simulink model "quadrotor_modules"  (R2020b)
settings: Solver=VariableStepAuto  StartTime=0.0  StopTime=10.0  RelTol=1e-3
values from neighbouring files (symbols this model uses):
  b = 1    [quadrotor_parameters.m]
  d = 1    [quadrotor_parameters.m]
  g = 9.81    [quadrotor_parameters.m]
  Ix = 1    [quadrotor_parameters.m]
  Iy = 1    [quadrotor_parameters.m]
  Iz = 1.5    [quadrotor_parameters.m]
  l = 1    [quadrotor_parameters.m]
  m = 1    [quadrotor_parameters.m]
settings Model: Creator=Алексей  LastModifiedBy=Алексей

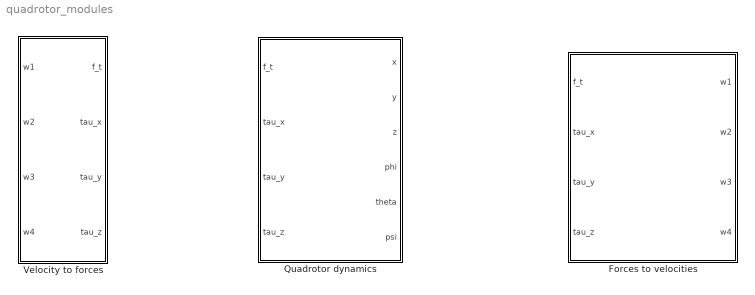
== system quadrotor_modules ==
  Forces to velocities : Subsystem
  Quadrotor dynamics : Subsystem
  Velocity to forces : Subsystem

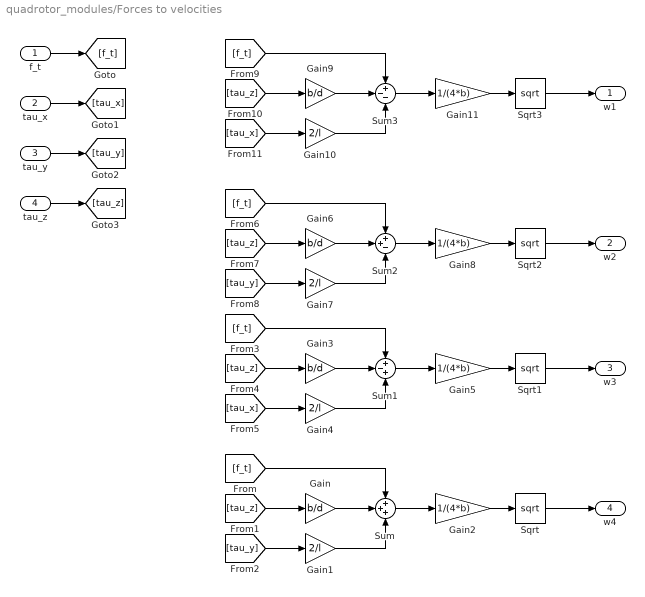
== system quadrotor_modules/Forces to velocities ==
  f_t : Inport
  tau_x : Inport  Port=2
  tau_y : Inport  Port=3
  tau_z : Inport  Port=4
  Gain{,3,6,9} (4 alike) : Gain  Gain=b/d
  Gain{1,4,7,10} (4 alike) : Gain  Gain=2/l
  Gain{2,5,8,11} (4 alike) : Gain  Gain=1/(4*b)
  Sqrt{,1..3} (4 alike) : Sqrt  SaturateOnIntegerOverflow=on
  Sum : Sum  Inputs=+++
  Sum1 : Sum  Inputs=+-+
  Sum2 : Sum  Inputs=++-
  Sum3 : Sum  Inputs=+--
  w1 : Outport
  w2 : Outport  Port=2
  w3 : Outport  Port=3
  w4 : Outport  Port=4
  wires:
  f_t/1 -> [f_t]
  [tau_y] -> Gain1/1
  [f_t] -> Sum/1
  Gain2/1 -> Sqrt/1
  Sqrt/1 -> w4/1
  Sum/1 -> Gain2/1
  tau_x/1 -> [tau_x]
  Gain/1 -> Sum/2
  Gain1/1 -> Sum/3
  tau_z/1 -> [tau_z]
  tau_y/1 -> [tau_y]
  [tau_z] -> Gain/1
  [tau_z] -> Gain3/1
  Gain4/1 -> Sum1/3
  Gain3/1 -> Sum1/2
  Sum1/1 -> Gain5/1
  Sqrt1/1 -> w3/1
  Gain5/1 -> Sqrt1/1
  [f_t] -> Sum1/1
  [tau_x] -> Gain4/1
  [tau_y] -> Gain7/1
  [f_t] -> Sum2/1
  Gain8/1 -> Sqrt2/1
  Sqrt2/1 -> w2/1
  Sum2/1 -> Gain8/1
  Gain6/1 -> Sum2/2
  Gain7/1 -> Sum2/3
  [tau_z] -> Gain6/1
  [tau_z] -> Gain9/1
  Gain10/1 -> Sum3/3
  Gain9/1 -> Sum3/2
  Sum3/1 -> Gain11/1
  Sqrt3/1 -> w1/1
  Gain11/1 -> Sqrt3/1
  [f_t] -> Sum3/1
  [tau_x] -> Gain10/1

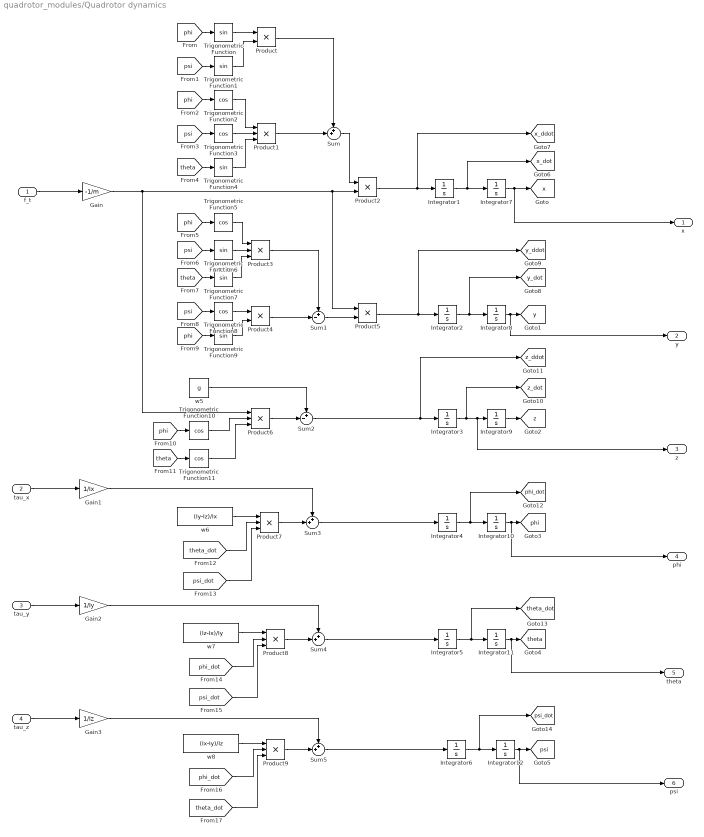
== system quadrotor_modules/Quadrotor dynamics ==
  f_t : Inport
  tau_x : Inport  Port=2
  tau_y : Inport  Port=3
  tau_z : Inport  Port=4
  Gain : Gain  Gain=-1/m
  Gain1 : Gain  Gain=1/Ix
  Gain2 : Gain  Gain=1/Iy
  Gain3 : Gain  Gain=1/Iz
  Integrator{1..12} (12 alike) : Integrator
  Product{,2,4..5} (4 alike) : Product
  Product{1,3,6..9} (6 alike) : Product  Inputs=3
  Sum{,3..5} (4 alike) : Sum  Inputs=++|
  Sum1 : Sum  Inputs=+-|
  Sum2 : Sum  Inputs=+-|
  Trigonometric Function{,1,4,6..7,9} (6 alike) : Trigonometry
  Trigonometric Function{2..3,5,8,10..11} (6 alike) : Trigonometry  Operator=cos
  w5 : Constant  Value=g
  w6 : Constant  Value=(Iy-Iz)/Ix
  w7 : Constant  Value=(Iz-Ix)/Iy
  w8 : Constant  Value=(Ix-Iy)/Iz
  x : Outport
  y : Outport  Port=2
  z : Outport  Port=3
  phi : Outport  Port=4
  theta : Outport  Port=5
  psi : Outport  Port=6
  tag scope: phi=global, phi_dot=global, psi=global, psi_dot=global, theta=global, theta_dot=global, x=global, x_ddot=global, x_dot=global, y=global, y_ddot=global, y_dot=global, z=global, z_ddot=global, z_dot=global
  wires:
  Integrator2/1 -> Integrator8/1, [y_dot]
  [theta_dot] -> Product9/3
  Integrator6/1 -> Integrator12/1, [psi_dot]
  Trigonometric Function4/1 -> Product1/3
  Trigonometric Function6/1 -> Product3/2
  tau_x/1 -> Gain1/1
  Product4/1 -> Sum1/2
  Trigonometric Function8/1 -> Product4/1
  Product2/1 -> [x_ddot], Integrator1/1
  [psi_dot] -> Product8/3
  Product/1 -> Sum/1
  [psi] -> Trigonometric Function6/1
  Product3/1 -> Sum1/1
  [psi] -> Trigonometric Function1/1
  Trigonometric Function1/1 -> Product/2
  Integrator4/1 -> Integrator10/1, [phi_dot]
  Integrator10/1 -> phi/1, [phi]
  Sum1/1 -> Product5/2
  Trigonometric Function5/1 -> Product3/1
  w6/1 -> Product7/1
  Trigonometric Function7/1 -> Product3/3
  Integrator3/1 -> [z_dot], z/1, Integrator9/1
  Trigonometric Function10/1 -> Product6/2
  [phi] -> Trigonometric Function5/1
  [phi] -> Trigonometric Function2/1
  Sum5/1 -> Integrator6/1
  Sum2/1 -> [z_ddot], Integrator3/1
  [phi_dot] -> Product8/2
  Integrator9/1 -> [z]
  Trigonometric Function3/1 -> Product1/2
  Integrator5/1 -> Integrator11/1, [theta_dot]
  Integrator12/1 -> psi/1, [psi]
  Product6/1 -> Sum2/2
  Product1/1 -> Sum/2
  Integrator1/1 -> Integrator7/1, [x_dot]
  f_t/1 -> Gain/1
  w5/1 -> Sum2/1
  [theta] -> Trigonometric Function7/1
  Product7/1 -> Sum3/2
  [phi] -> Trigonometric Function10/1
  Product5/1 -> [y_ddot], Integrator2/1
  [psi] -> Trigonometric Function8/1
  Trigonometric Function2/1 -> Product1/1
  [psi] -> Trigonometric Function3/1
  Trigonometric Function9/1 -> Product4/2
  [phi] -> Trigonometric Function/1
  Sum/1 -> Product2/1
  Integrator7/1 -> x/1, [x]
  Sum3/1 -> Integrator4/1
  [theta] -> Trigonometric Function4/1
  [psi_dot] -> Product7/3
  [theta] -> Trigonometric Function11/1
  [phi] -> Trigonometric Function9/1
  Integrator11/1 -> theta/1, [theta]
  Product9/1 -> Sum5/2
  [phi_dot] -> Product9/2
  Product8/1 -> Sum4/2
  Trigonometric Function11/1 -> Product6/3
  w8/1 -> Product9/1
  Integrator8/1 -> y/1, [y]
  [theta_dot] -> Product7/2
  Sum4/1 -> Integrator5/1
  Trigonometric Function/1 -> Product/1
  w7/1 -> Product8/1
  tau_z/1 -> Gain3/1
  tau_y/1 -> Gain2/1
  Gain/1 -> Product6/1, Product5/1, Product2/2
  Gain1/1 -> Sum3/1
  Gain2/1 -> Sum4/1
  Gain3/1 -> Sum5/1

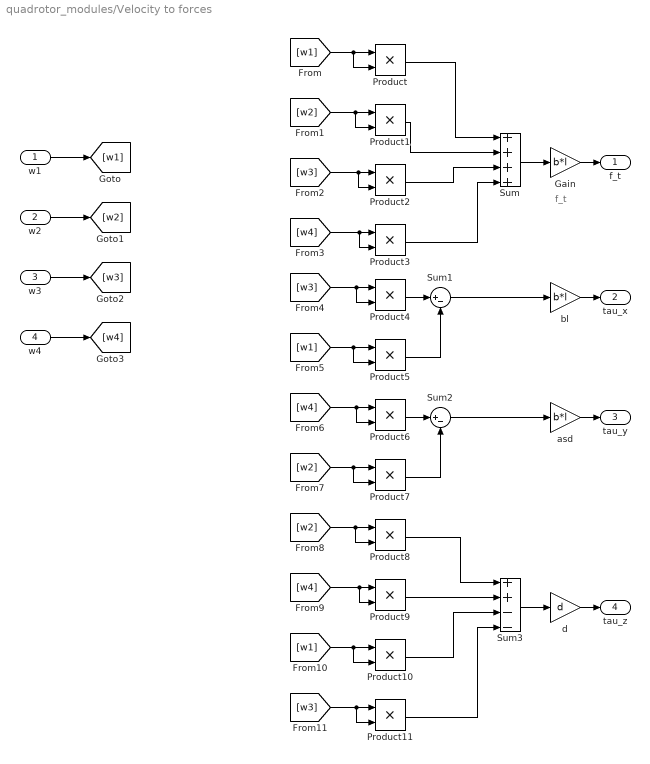
== system quadrotor_modules/Velocity to forces ==
  note: f_t
  w1 : Inport
  w2 : Inport  Port=2
  w3 : Inport  Port=3
  w4 : Inport  Port=4
  Gain : Gain  Gain=b*l
  Product{,1..11} (12 alike) : Product
  Sum : Sum  Inputs=++++
  Sum1 : Sum  Inputs=|+-
  Sum2 : Sum  Inputs=|+-
  Sum3 : Sum  Inputs=++--
  asd : Gain  Gain=b*l
  bl : Gain  Gain=b*l
  d : Gain  Gain=d
  f_t : Outport
  tau_x : Outport  Port=2
  tau_y : Outport  Port=3
  tau_z : Outport  Port=4
  wires:
  Product4/1 -> Sum1/1
  Product9/1 -> Sum3/2
  [w1] -> Product10/1, Product10/2
  Product11/1 -> Sum3/4
  Product2/1 -> Sum/3
  d/1 -> tau_z/1
  [w3] -> Product2/2, Product2/1
  [w2] -> Product1/2, Product1/1
  [w1] -> Product/2, Product/1
  [w2] -> Product8/1, Product8/2
  w3/1 -> [w3]
  [w3] -> Product4/2, Product4/1
  Product10/1 -> Sum3/3
  [w1] -> Product5/1, Product5/2
  Product5/1 -> Sum1/2
  [w3] -> Product11/1, Product11/2
  [w2] -> Product7/2, Product7/1
  Product/1 -> Sum/1
  Product6/1 -> Sum2/1
  Product8/1 -> Sum3/1
  bl/1 -> tau_x/1
  [w4] -> Product9/1, Product9/2
  Sum2/1 -> asd/1
  [w4] -> Product3/2, Product3/1
  w2/1 -> [w2]
  Product1/1 -> Sum/2
  Gain/1 -> f_t/1
  Product7/1 -> Sum2/2
  [w4] -> Product6/1, Product6/2
  asd/1 -> tau_y/1
  w1/1 -> [w1]
  Product3/1 -> Sum/4
  w4/1 -> [w4]
  Sum3/1 -> d/1
  Sum1/1 -> bl/1
  Sum/1 -> Gain/1
